simulink model "PMSM_Simulation"  (R2023a)
settings: Solver=ode23t  StartTime=0.0  StopTime=5  MaxStep=0.2  RelTol=1e-4  EnableMultiTasking=on
InitFcn:
  | p = 4;
  | Ld = 0.000425;
  | Lq = 0.00085;
  | psim = 0.119489;
  | Rs = 0.0485;
  | J = 0.00027;
  | Kpwm = 1;
  | Tsi = 0.0001;
  | h = 900;
  | 
  | L0 = (Ld+Lq)/2;
  | SMO_Kp = 100;
  | SMO_Coef =0.0001;
  | Ki_id = Ld*(h+1)/(4.5*Kpwm*(Tsi^2)*(h^2));
  | Kp_id = Ld*(h+1)/(4.5*Kpwm*Tsi*h);
  | 
  | wc =3000;
  | 
  | Ki_iq = Lq*(h+1)/(4.5*Kpwm*Tsi^2*h^2);
  | Kp_iq = Lq*(h+1)/(4.5*Kpwm*Tsi*h);
  | 
  | 
  | Kp_Spd = pi*J/(300*p*psim*Tsi)
  | Ki_Spd = pi*J/(6000*p*psim*Tsi^2)
  | 
  | DeadTime = 2e-6;
  | 
  | Udc = 650;
model workspace (MAT data in the model file):
  KfDeadCompen_CpPeriodTimesT_NULL : Simulink.Parameter (value not decoded)
  KfMDCC_InvParkCpPeriodTimesT_NULL : Simulink.Parameter (value not decoded)
values from neighbouring files (symbols this model uses):
  KfDeadCompen_SetDeltaTime_us = myPackage.Parameter    [DeadCompen.m]
  VbDeadComp_SwtUseIsttrDes_flg = myPackage.Parameter    [DeadCompen.m]
  VfDeadCompen_agIPredAdpr_C = myPackage.Parameter    [DeadCompen.m]
  VfDeadCompen_ISttrDdeThdSwt_A = myPackage.Parameter    [DeadCompen.m]
  VfDeadCompen_ISttrIgbtThdSwt_A = myPackage.Parameter    [DeadCompen.m]
  VfDeadCompen_rDdeISttrHi_R = myPackage.Parameter    [DeadCompen.m]
  VfDeadCompen_rDdeISttrLo_R = myPackage.Parameter    [DeadCompen.m]
  VfDeadCompen_rIgbtISttrHi_R = myPackage.Parameter    [DeadCompen.m]
  VfDeadCompen_rIgbtISttrLo_R = myPackage.Parameter    [DeadCompen.m]
  VfDeadCompen_uDdeISttrHi_V = myPackage.Parameter    [DeadCompen.m]
  VfDeadCompen_uDdeISttrLo_V = myPackage.Parameter    [DeadCompen.m]
  VfDeadCompen_uIgbtISttrHi_V = myPackage.Parameter    [DeadCompen.m]
  VfDeadCompen_uIgbtISttrLo_V = myPackage.Parameter    [DeadCompen.m]
symbols that are objects in the model workspace (value not decoded): KfDeadCompen_CpPeriodTimesT_NULL, KfMDCC_InvParkCpPeriodTimesT_NULL
undefined symbols (not defined in the file or in its folder): DiscIntNeverNeededParam, TableDeadTime_us, TableDeadTimeLookUpCur_A, VuDeadCompen_agIPredAdpr_C
libraries: simulink x23, mcbcontrolslib x11, mcbplantlib x1, spsCurrentMeasurementLib x1, spsDCVoltageSourceLib x1, spsMultimeterLib x1, spsPermanentMagnetSynchronousMachineLib x1, eePmsmCurrentController x1, spsThreePhaseVIMeasurementLib x1, spsUniversalBridgeLib x1, spspowerguiLib x1
(part 3 of 4)

== system PMSM_Simulation/Subsystem/Subsystem/Subsystem2/Subsystem2/Subsystem3 ==
  eMtrSpd_rads : Inport
  eMtrPos_NULL : Inport  Port=2
  VfPwmFreq_Hz : Inport  Port=3
  Isd_A : Inport  Port=4
  Isq_A : Inport  Port=5
  Add : Sum  Inputs=+++
  Constant2 : Constant  Value=2*pi  OutDataTypeStr=single
  Constant3 : Constant  Value=pi/6  OutDataTypeStr=single
  Constant4 : Constant  Value=pi/3  OutDataTypeStr=single
  Data Type Conversion : DataTypeConversion  OutDataTypeStr=uint8  SaturateOnIntegerOverflow=off  RndMeth=Floor
  Divide : Product  Inputs=*/
  Mod : Math  Operator=mod
  Subsystem1 : Subsystem
  Subsystem2 : Subsystem
  PreMtrPos : Outport
  Select_N : Outport  Port=2
  wires:
  Constant3/1 -> Add/3
  Mod/1 -> Divide/1
  Subsystem2/1(PreMtrPos) -> PreMtrPos/1, Add/1
  Constant2/1 -> Mod/2
  eMtrPos_NULL/1 -> Subsystem2/2(eMtrPos_NULL)
  Add/1 -> Mod/1
  Subsystem1/1(agIsE) -> Add/2
  Divide/1 -> Data Type Conversion/1
  Constant4/1 -> Divide/2
  Data Type Conversion/1 -> Select_N/1
  Isq_A/1 -> Subsystem1/2(Isq_A)
  Isd_A/1 -> Subsystem1/1(Isd_A)
  VfPwmFreq_Hz/1 -> Subsystem2/3(VfPwmFreq_Hz)
  eMtrSpd_rads/1 -> Subsystem2/1(eMtrSpd_rads)

== system PMSM_Simulation/Subsystem/Subsystem/Subsystem4/Subsystem1/Subsystem ==
  In1 : Inport
  Compare To Constant : simulink/Logic and Bit Operations/Compare To Constant  relop=>=  const=0  OutDataTypeStr=boolean
  Constant1 : Constant  Value=0
  Switch : Switch  Criteria=u2 > Threshold  SaturateOnIntegerOverflow=off  InputSameDT=off
  Out1 : Outport
  wires:
  In1/1 -> Switch/1, Compare To Constant/1
  Constant1/1 -> Switch/3
  Compare To Constant/1 -> Switch/2
  Switch/1 -> Out1/1

== system PMSM_Simulation/Subsystem/Subsystem/Subsystem4/Subsystem2/Subsystem ==
  In1 : Inport
  Compare To Constant : simulink/Logic and Bit Operations/Compare To Constant  relop=>=  const=0  OutDataTypeStr=boolean
  Constant1 : Constant  Value=0
  Switch : Switch  Criteria=u2 > Threshold  SaturateOnIntegerOverflow=off  InputSameDT=off
  Out1 : Outport
  wires:
  In1/1 -> Switch/1, Compare To Constant/1
  Constant1/1 -> Switch/3
  Compare To Constant/1 -> Switch/2
  Switch/1 -> Out1/1

== system PMSM_Simulation/Subsystem/Subsystem/Subsystem4/Subsystem3/Subsystem ==
  In1 : Inport
  Compare To Constant : simulink/Logic and Bit Operations/Compare To Constant  relop=>=  const=0  OutDataTypeStr=boolean
  Constant1 : Constant  Value=0
  Switch : Switch  Criteria=u2 > Threshold  SaturateOnIntegerOverflow=off  InputSameDT=off
  Out1 : Outport
  wires:
  In1/1 -> Switch/1, Compare To Constant/1
  Constant1/1 -> Switch/3
  Compare To Constant/1 -> Switch/2
  Switch/1 -> Out1/1

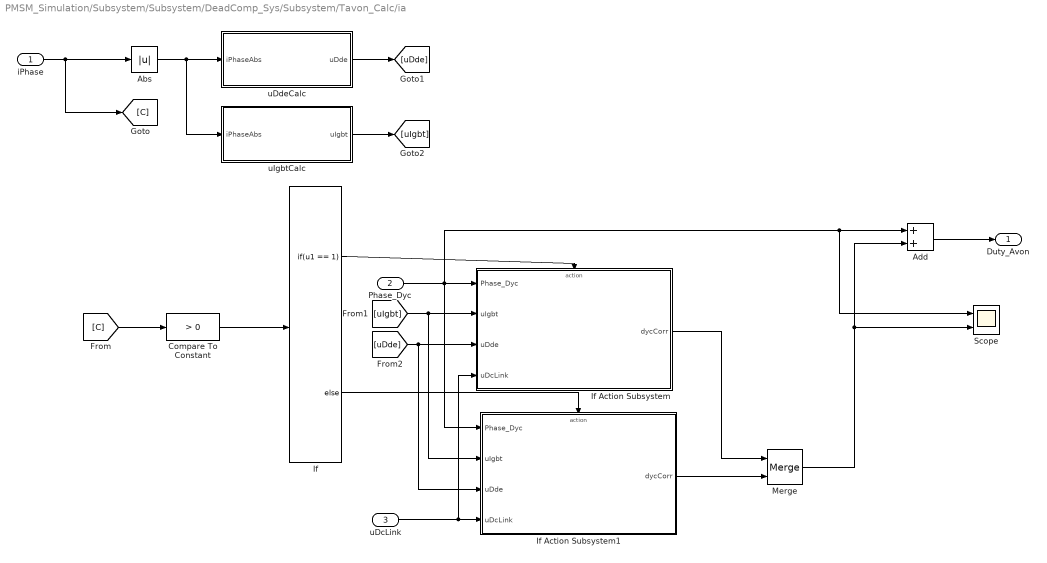
== system PMSM_Simulation/Subsystem/Subsystem/DeadComp_Sys/Subsystem/Tavon_Calc/ia ==
  iPhase : Inport
  Phase_Dyc : Inport  Port=2
  uDcLink : Inport  Port=3
  Abs : Abs  SaturateOnIntegerOverflow=off
  Add : Sum
  Compare To Constant : simulink/Logic and Bit Operations/Compare To Constant  relop=>  const=0  OutDataTypeStr=boolean
  If : If  IfExpression=u1 == 1
  If Action Subsystem : Subsystem  TreatAsAtomicUnit=on
  If Action Subsystem1 : Subsystem  TreatAsAtomicUnit=on
  Merge : Merge
  Scope : Scope  NumInputPorts=2
  uDdeCalc : Subsystem
  uIgbtCalc : Subsystem
  "Duty_Avon " : Outport
  wires:
  iPhase/1 -> [C], Abs/1
  Abs/1 -> uIgbtCalc/1(iPhaseAbs), uDdeCalc/1(iPhaseAbs)
  uDdeCalc/1(uDde) -> [uDde]
  uIgbtCalc/1(uIgbt) -> [uIgbt]
  [C] -> Compare To Constant/1
  Compare To Constant/1 -> If/1
  If/1 -> If Action Subsystem/Action
  If/2 -> If Action Subsystem1/Action
  [uIgbt] -> If Action Subsystem1/2(uIgbt), If Action Subsystem/2(uIgbt)
  [uDde] -> If Action Subsystem1/3(uDde), If Action Subsystem/3(uDde)
  Phase_Dyc/1 -> Scope/1, Add/1, If Action Subsystem1/1(Phase_Dyc), If Action Subsystem/1(Phase_Dyc)
  uDcLink/1 -> If Action Subsystem/4(uDcLink), If Action Subsystem1/4(uDcLink)
  If Action Subsystem1/1("dycCorr ") -> Merge/2
  If Action Subsystem/1("dycCorr ") -> Merge/1
  Add/1 -> "Duty_Avon "/1
  Merge/1 -> Scope/2, Add/2

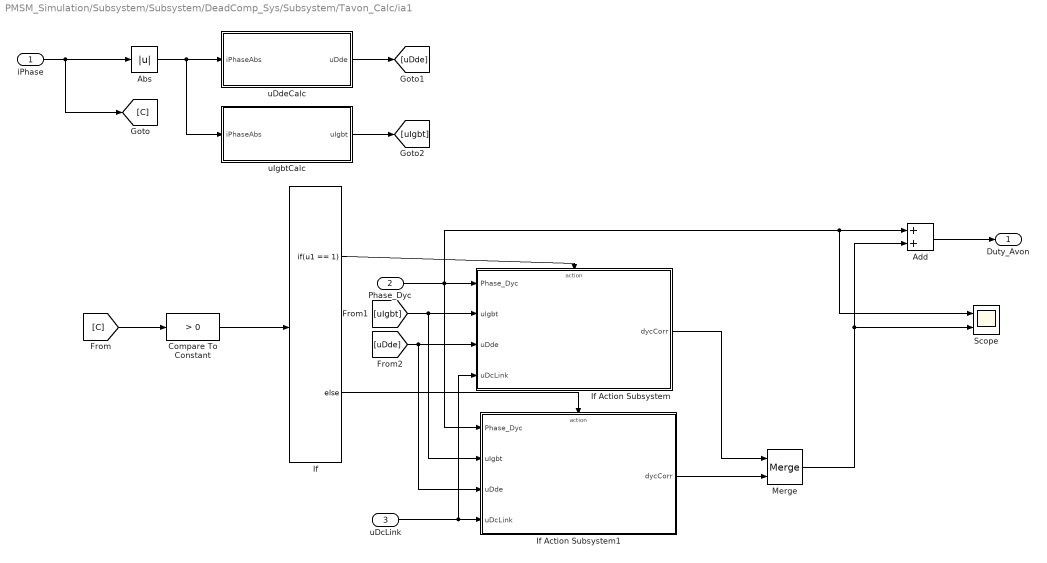
== system PMSM_Simulation/Subsystem/Subsystem/DeadComp_Sys/Subsystem/Tavon_Calc/ia1 ==
  iPhase : Inport
  Phase_Dyc : Inport  Port=2
  uDcLink : Inport  Port=3
  Abs : Abs  SaturateOnIntegerOverflow=off
  Add : Sum
  Compare To Constant : simulink/Logic and Bit Operations/Compare To Constant  relop=>  const=0  OutDataTypeStr=boolean
  If : If  IfExpression=u1 == 1
  If Action Subsystem : Subsystem  TreatAsAtomicUnit=on
  If Action Subsystem1 : Subsystem  TreatAsAtomicUnit=on
  Merge : Merge
  Scope : Scope  NumInputPorts=2
  uDdeCalc : Subsystem
  uIgbtCalc : Subsystem
  "Duty_Avon " : Outport
  wires:
  iPhase/1 -> [C], Abs/1
  Abs/1 -> uIgbtCalc/1(iPhaseAbs), uDdeCalc/1(iPhaseAbs)
  uDdeCalc/1(uDde) -> [uDde]
  uIgbtCalc/1(uIgbt) -> [uIgbt]
  [C] -> Compare To Constant/1
  Compare To Constant/1 -> If/1
  If/1 -> If Action Subsystem/Action
  If/2 -> If Action Subsystem1/Action
  [uIgbt] -> If Action Subsystem1/2(uIgbt), If Action Subsystem/2(uIgbt)
  [uDde] -> If Action Subsystem1/3(uDde), If Action Subsystem/3(uDde)
  Phase_Dyc/1 -> Scope/1, Add/1, If Action Subsystem1/1(Phase_Dyc), If Action Subsystem/1(Phase_Dyc)
  uDcLink/1 -> If Action Subsystem/4(uDcLink), If Action Subsystem1/4(uDcLink)
  If Action Subsystem1/1("dycCorr ") -> Merge/2
  If Action Subsystem/1("dycCorr ") -> Merge/1
  Add/1 -> "Duty_Avon "/1
  Merge/1 -> Scope/2, Add/2

== system PMSM_Simulation/Subsystem/Subsystem/DeadComp_Sys/Subsystem/Tavon_Calc/ia2 ==
  iPhase : Inport
  Phase_Dyc : Inport  Port=2
  uDcLink : Inport  Port=3
  Abs : Abs  SaturateOnIntegerOverflow=off
  Add : Sum
  Compare To Constant : simulink/Logic and Bit Operations/Compare To Constant  relop=>  const=0  OutDataTypeStr=boolean
  If : If  IfExpression=u1 == 1
  If Action Subsystem : Subsystem  TreatAsAtomicUnit=on
  If Action Subsystem1 : Subsystem  TreatAsAtomicUnit=on
  Merge : Merge
  Scope : Scope  NumInputPorts=2
  uDdeCalc : Subsystem
  uIgbtCalc : Subsystem
  "Duty_Avon " : Outport
  wires:
  iPhase/1 -> [C], Abs/1
  Abs/1 -> uIgbtCalc/1(iPhaseAbs), uDdeCalc/1(iPhaseAbs)
  uDdeCalc/1(uDde) -> [uDde]
  uIgbtCalc/1(uIgbt) -> [uIgbt]
  [C] -> Compare To Constant/1
  Compare To Constant/1 -> If/1
  If/1 -> If Action Subsystem/Action
  If/2 -> If Action Subsystem1/Action
  [uIgbt] -> If Action Subsystem1/2(uIgbt), If Action Subsystem/2(uIgbt)
  [uDde] -> If Action Subsystem1/3(uDde), If Action Subsystem/3(uDde)
  Phase_Dyc/1 -> Scope/1, Add/1, If Action Subsystem1/1(Phase_Dyc), If Action Subsystem/1(Phase_Dyc)
  uDcLink/1 -> If Action Subsystem/4(uDcLink), If Action Subsystem1/4(uDcLink)
  If Action Subsystem1/1("dycCorr ") -> Merge/2
  If Action Subsystem/1("dycCorr ") -> Merge/1
  Add/1 -> "Duty_Avon "/1
  Merge/1 -> Scope/2, Add/2

== system PMSM_Simulation/Subsystem/Subsystem/DeadComp_Sys/Subsystem2/Subsystem3/Subsystem1 ==
  Isd_A : Inport
  Isq_A : Inport  Port=2
  Add : Sum
  Atan2 : Trigonometry  Operator=atan2
  Constant : Constant  Value=2*pi  OutDataTypeStr=single
  Switch : Switch  Criteria=u2 > Threshold  SaturateOnIntegerOverflow=off  InputSameDT=off
  agIsE : Outport
  wires:
  Isd_A/1 -> Atan2/2
  Isq_A/1 -> Atan2/1
  Atan2/1 -> Add/1, Switch/1, Switch/2
  Switch/1 -> agIsE/1
  Add/1 -> Switch/3
  Constant/1 -> Add/2

== system PMSM_Simulation/Subsystem/Subsystem/DeadComp_Sys/Subsystem2/Subsystem3/Subsystem2 ==
  eMtrSpd_rads : Inport
  eMtrPos_NULL : Inport  Port=2
  VfPwmFreq_Hz : Inport  Port=3
  Add : Sum  Inputs=+++
  Constant : Constant  Value=VuDeadCompen_agIPredAdpr_C
  Gain : Gain  Gain=2*pi/4095
  Gain1 : Gain  Gain=-1
  Gain2 : Gain  Gain=2*pi/4095
  Product : Product
  Subsystem : Subsystem
  Switch : Switch  Criteria=u2 > Threshold  SaturateOnIntegerOverflow=off  InputSameDT=off
  PreMtrPos : Outport
  wires:
  VfPwmFreq_Hz/1 -> Subsystem/1(VfPwmFreq_Hz)
  Subsystem/1(TimeComp) -> Product/2
  eMtrPos_NULL/1 -> Gain/1
  Product/1 -> Add/2
  Gain/1 -> Add/3
  Add/1 -> PreMtrPos/1
  eMtrSpd_rads/1 -> Product/1, Switch/2
  Constant/1 -> Gain2/1
  Gain1/1 -> Switch/3
  Gain2/1 -> Gain1/1, Switch/1
  Switch/1 -> Add/1

== system PMSM_Simulation/Subsystem/Subsystem/SVM_PU/T1_T2_Calc/Subsystem1/Enabled Subsystem ==
  Z : Inport
  Y : Inport  Port=2
  Action Port : ActionPort  ActionPortLabel=case [ 1 ]:
  T4 : Outport
  T6 : Outport  Port=2
  wires:
  Z/1 -> T4/1
  Y/1 -> T6/1

== system PMSM_Simulation/Subsystem/Subsystem/SVM_PU/T1_T2_Calc/Subsystem1/Enabled Subsystem1 ==
  Y : Inport
  X : Inport  Port=2
  Action Port : ActionPort  ActionPortLabel=case [ 2 ]:
  Gain : Gain  Gain=-1
  T4 : Outport
  T6 : Outport  Port=2
  wires:
  Y/1 -> T4/1
  Gain/1 -> T6/1
  X/1 -> Gain/1

== system PMSM_Simulation/Subsystem/Subsystem/SVM_PU/T1_T2_Calc/Subsystem1/Enabled Subsystem2 ==
  Z : Inport
  X : Inport  Port=2
  Action Port : ActionPort  ActionPortLabel=case [ 3 ]:
  Gain : Gain  Gain=-1
  T4 : Outport
  T6 : Outport  Port=2
  wires:
  Z/1 -> Gain/1
  X/1 -> T6/1
  Gain/1 -> T4/1

== system PMSM_Simulation/Subsystem/Subsystem/SVM_PU/T1_T2_Calc/Subsystem1/Enabled Subsystem3 ==
  X : Inport
  Z : Inport  Port=2
  Action Port : ActionPort  ActionPortLabel=case [ 4 ]:
  Gain : Gain  Gain=-1
  T4 : Outport
  T6 : Outport  Port=2
  wires:
  X/1 -> Gain/1
  Z/1 -> T6/1
  Gain/1 -> T4/1

== system PMSM_Simulation/Subsystem/Subsystem/SVM_PU/T1_T2_Calc/Subsystem1/Enabled Subsystem4 ==
  X : Inport
  Y : Inport  Port=2
  Action Port : ActionPort  ActionPortLabel=case [ 5 ]:
  Gain : Gain  Gain=-1
  T4 : Outport
  T6 : Outport  Port=2
  wires:
  Y/1 -> Gain/1
  X/1 -> T4/1
  Gain/1 -> T6/1

== system PMSM_Simulation/Subsystem/Subsystem/SVM_PU/T1_T2_Calc/Subsystem1/Enabled Subsystem5 ==
  Y : Inport
  Z : Inport  Port=2
  Action Port : ActionPort  ActionPortLabel=case [ 6 ]:
  Gain : Gain  Gain=-1
  Gain1 : Gain  Gain=-1
  T4 : Outport
  T6 : Outport  Port=2
  wires:
  Y/1 -> Gain/1
  Z/1 -> Gain1/1
  Gain/1 -> T4/1
  Gain1/1 -> T6/1

== system PMSM_Simulation/Subsystem/Subsystem/SVM_PU/T1_T2_Calc/Subsystem1/Enabled Subsystem6 ==
  Y : Inport
  Z : Inport  Port=2
  Action Port : ActionPort  ActionPortLabel=default:
  Gain : Gain  Gain=-1
  Gain1 : Gain  Gain=-1
  T4 : Outport
  T6 : Outport  Port=2
  wires:
  Y/1 -> Gain/1
  Z/1 -> Gain1/1
  Gain/1 -> T4/1
  Gain1/1 -> T6/1

== system PMSM_Simulation/Subsystem/Subsystem/SVM_PU/T1_T2_Calc/Subsystem2/If Action Subsystem ==
  Bus_T4T6 : Inport
  Action Port : ActionPort  ActionPortLabel=else
  Bus Selector : BusSelector  OutputSignals=T4,T6
  Signal Copy1 : SignalConversion  OverrideOpt=off
  Signal Copy2 : SignalConversion  OverrideOpt=off
  T1 : Outport
  T2 : Outport  Port=2
  wires:
  Bus_T4T6/1 -> Bus Selector/1
  Bus Selector/1 -> Signal Copy1/1  "<T4>"
  Bus Selector/2 -> Signal Copy2/1  "<T6>"
  Signal Copy1/1 -> T1/1
  Signal Copy2/1 -> T2/1

== system PMSM_Simulation/Subsystem/Subsystem/SVM_PU/T1_T2_Calc/Subsystem2/If Action Subsystem1 ==
  Bus_T4T6 : Inport
  Action Port : ActionPort  ActionPortLabel=elseif(u1 > 1)
  Add : Sum
  Bus Selector : BusSelector  OutputSignals=T4,T6
  Divide : Product  Inputs=*/
  Divide1 : Product  Inputs=/*
  T1 : Outport
  T2 : Outport  Port=2
  wires:
  Bus_T4T6/1 -> Bus Selector/1
  Bus Selector/1 -> Divide/1, Add/1  "<T4>"
  Bus Selector/2 -> Divide1/2, Add/2  "<T6>"
  Add/1 -> Divide1/1, Divide/2
  Divide/1 -> T1/1  "T1"
  Divide1/1 -> T2/1  "T2"

== system PMSM_Simulation/Subsystem/Subsystem/SVM_PU/T1_T2_Calc/Subsystem2/If Action Subsystem2 ==
  Bus_T4T6 : Inport
  Action Port : ActionPort  ActionPortLabel=if(u1 > 1.154 )
  Add1 : Sum
  Add2 : Sum  Inputs=++-
  Bus Selector1 : BusSelector  OutputSignals=T4,T6
  Constant : Constant  Value=1.154  OutDataTypeStr=single
  Divide : Product  Inputs=*/
  Divide1 : Product  Inputs=/*
  If Action Subsystem2 : Subsystem  TreatAsAtomicUnit=on
  If Action Subsystem3 : Subsystem  TreatAsAtomicUnit=on
  If1 : If  IfExpression=u1 ~= 0
  Merge2 : Merge
  Merge3 : Merge
  Relational Operator1 : RelationalOperator  OutDataTypeStr=boolean  RndMeth=Simplest  InputSameDT=off
  T1 : Outport
  T2 : Outport  Port=2
  wires:
  Bus_T4T6/1 -> Bus Selector1/1
  Bus Selector1/2 -> Divide1/2, Add2/2, Add1/2  "<T6>"
  Divide/1 -> [T4_m], Relational Operator1/1  "T4_m"
  Bus Selector1/1 -> Divide/1, Add2/1, Add1/1  "<T4>"
  Divide1/1 -> [T6_m], Relational Operator1/2  "T6_m"
  Add1/1 -> Divide1/1, Divide/2
  Relational Operator1/1 -> If1/1
  Constant/1 -> Add2/3
  Add2/1 -> If Action Subsystem2/3(delta), If Action Subsystem3/3(delta)  "delta"
  If1/1 -> If Action Subsystem2/Action
  If1/2 -> If Action Subsystem3/Action
  If Action Subsystem2/1(T1) -> Merge2/1
  If Action Subsystem3/1(T1) -> Merge2/2
  If Action Subsystem3/2(T2) -> Merge3/2
  If Action Subsystem2/2(T2) -> Merge3/1
  Merge2/1 -> T1/1  "T1"
  Merge3/1 -> T2/1  "T2"
  [T4_m] -> If Action Subsystem3/1(T4_m), If Action Subsystem2/1(T4_m)
  [T6_m] -> If Action Subsystem3/2(T6_m), If Action Subsystem2/2(T6_m)

== system PMSM_Simulation/Subsystem/Subsystem/Subsystem2/Subsystem/DutyErr_Calc/PhaseU ==
  Bus_DutyAvon : Inport
  Bus_DeltaTimeOnOffDuty : Inport  Port=2
  DeadTimeDuty : Inport  Port=3
  Add : Sum  Inputs=+-+
  Bus Selector : BusSelector  OutputSignals=DutyAvon_U
  Bus Selector1 : BusSelector  OutputSignals=DeltaTimeOnOffU_NULL
  DutyCompensate_U : Outport
  wires:
  Bus_DutyAvon/1 -> Bus Selector/1
  Bus_DeltaTimeOnOffDuty/1 -> Bus Selector1/1
  Bus Selector1/1 -> Add/2  "<DeltaTimeOnOffU_NULL>"
  Bus Selector/1 -> Add/1  "<DutyAvon_U>"
  DeadTimeDuty/1 -> Add/3
  Add/1 -> DutyCompensate_U/1

== system PMSM_Simulation/Subsystem/Subsystem/Subsystem2/Subsystem/DutyErr_Calc/PhaseV ==
  Bus_DutyAvon : Inport
  Bus_DeltaTimeOnOffDuty : Inport  Port=2
  DeadTimeDuty : Inport  Port=3
  Add : Sum  Inputs=+++
  Bus Selector : BusSelector  OutputSignals=DutyAvon_V
  Bus Selector1 : BusSelector  OutputSignals=DeltaTimeOnOffV_NULL
  DutyCompensate_V : Outport
  wires:
  Bus_DutyAvon/1 -> Bus Selector/1
  Bus_DeltaTimeOnOffDuty/1 -> Bus Selector1/1
  Bus Selector1/1 -> Add/2  "<DeltaTimeOnOffV_NULL>"
  Bus Selector/1 -> Add/1  "<DutyAvon_V>"
  DeadTimeDuty/1 -> Add/3
  Add/1 -> DutyCompensate_V/1

== system PMSM_Simulation/Subsystem/Subsystem/Subsystem2/Subsystem/DutyErr_Calc/PhaseW ==
  Bus_DutyAvon : Inport
  Bus_DeltaTimeOnOffDuty : Inport  Port=2
  DeadTimeDuty : Inport  Port=3
  Add : Sum  Inputs=+++
  Bus Selector : BusSelector  OutputSignals=DutyAvon_W
  Bus Selector1 : BusSelector  OutputSignals=DeltaTimeOnOffW_NULL
  DutyCompensate_W : Outport
  wires:
  Bus_DutyAvon/1 -> Bus Selector/1
  Bus_DeltaTimeOnOffDuty/1 -> Bus Selector1/1
  Bus Selector1/1 -> Add/2  "<DeltaTimeOnOffW_NULL>"
  Bus Selector/1 -> Add/1  "<DutyAvon_W>"
  DeadTimeDuty/1 -> Add/3
  Add/1 -> DutyCompensate_W/1

== system PMSM_Simulation/Subsystem/Subsystem/Subsystem2/Subsystem/Tavon_Calc/ia ==
  iPhase : Inport
  Phase_Dyc : Inport  Port=2
  uDcLink : Inport  Port=3
  Abs : Abs  SaturateOnIntegerOverflow=off
  Add : Sum
  Compare To Constant : simulink/Logic and Bit Operations/Compare To Constant  relop=>  const=0  OutDataTypeStr=boolean
  If : If  IfExpression=u1 == 1
  If Action Subsystem : Subsystem  TreatAsAtomicUnit=on
  If Action Subsystem1 : Subsystem  TreatAsAtomicUnit=on
  Merge : Merge
  Scope : Scope  NumInputPorts=2
  uDdeCalc : Subsystem
  uIgbtCalc : Subsystem
  "Duty_Avon " : Outport
  wires:
  iPhase/1 -> [C], Abs/1
  Abs/1 -> uIgbtCalc/1(iPhaseAbs), uDdeCalc/1(iPhaseAbs)
  uDdeCalc/1(uDde) -> [uDde]
  uIgbtCalc/1(uIgbt) -> [uIgbt]
  [C] -> Compare To Constant/1
  Compare To Constant/1 -> If/1
  If/1 -> If Action Subsystem/Action
  If/2 -> If Action Subsystem1/Action
  [uIgbt] -> If Action Subsystem1/2(uIgbt), If Action Subsystem/2(uIgbt)
  [uDde] -> If Action Subsystem1/3(uDde), If Action Subsystem/3(uDde)
  Phase_Dyc/1 -> Scope/1, Add/1, If Action Subsystem1/1(Phase_Dyc), If Action Subsystem/1(Phase_Dyc)
  uDcLink/1 -> If Action Subsystem/4(uDcLink), If Action Subsystem1/4(uDcLink)
  If Action Subsystem1/1("dycCorr ") -> Merge/2
  If Action Subsystem/1("dycCorr ") -> Merge/1
  Add/1 -> "Duty_Avon "/1
  Merge/1 -> Scope/2, Add/2

== system PMSM_Simulation/Subsystem/Subsystem/Subsystem2/Subsystem/Tavon_Calc/ia1 ==
  iPhase : Inport
  Phase_Dyc : Inport  Port=2
  uDcLink : Inport  Port=3
  Abs : Abs  SaturateOnIntegerOverflow=off
  Add : Sum
  Compare To Constant : simulink/Logic and Bit Operations/Compare To Constant  relop=>  const=0  OutDataTypeStr=boolean
  If : If  IfExpression=u1 == 1
  If Action Subsystem : Subsystem  TreatAsAtomicUnit=on
  If Action Subsystem1 : Subsystem  TreatAsAtomicUnit=on
  Merge : Merge
  Scope : Scope  NumInputPorts=2
  uDdeCalc : Subsystem
  uIgbtCalc : Subsystem
  "Duty_Avon " : Outport
  wires:
  iPhase/1 -> [C], Abs/1
  Abs/1 -> uIgbtCalc/1(iPhaseAbs), uDdeCalc/1(iPhaseAbs)
  uDdeCalc/1(uDde) -> [uDde]
  uIgbtCalc/1(uIgbt) -> [uIgbt]
  [C] -> Compare To Constant/1
  Compare To Constant/1 -> If/1
  If/1 -> If Action Subsystem/Action
  If/2 -> If Action Subsystem1/Action
  [uIgbt] -> If Action Subsystem1/2(uIgbt), If Action Subsystem/2(uIgbt)
  [uDde] -> If Action Subsystem1/3(uDde), If Action Subsystem/3(uDde)
  Phase_Dyc/1 -> Scope/1, Add/1, If Action Subsystem1/1(Phase_Dyc), If Action Subsystem/1(Phase_Dyc)
  uDcLink/1 -> If Action Subsystem/4(uDcLink), If Action Subsystem1/4(uDcLink)
  If Action Subsystem1/1("dycCorr ") -> Merge/2
  If Action Subsystem/1("dycCorr ") -> Merge/1
  Add/1 -> "Duty_Avon "/1
  Merge/1 -> Scope/2, Add/2

== system PMSM_Simulation/Subsystem/Subsystem/Subsystem2/Subsystem/Tavon_Calc/ia2 ==
  iPhase : Inport
  Phase_Dyc : Inport  Port=2
  uDcLink : Inport  Port=3
  Abs : Abs  SaturateOnIntegerOverflow=off
  Add : Sum
  Compare To Constant : simulink/Logic and Bit Operations/Compare To Constant  relop=>  const=0  OutDataTypeStr=boolean
  If : If  IfExpression=u1 == 1
  If Action Subsystem : Subsystem  TreatAsAtomicUnit=on
  If Action Subsystem1 : Subsystem  TreatAsAtomicUnit=on
  Merge : Merge
  Scope : Scope  NumInputPorts=2
  uDdeCalc : Subsystem
  uIgbtCalc : Subsystem
  "Duty_Avon " : Outport
  wires:
  iPhase/1 -> [C], Abs/1
  Abs/1 -> uIgbtCalc/1(iPhaseAbs), uDdeCalc/1(iPhaseAbs)
  uDdeCalc/1(uDde) -> [uDde]
  uIgbtCalc/1(uIgbt) -> [uIgbt]
  [C] -> Compare To Constant/1
  Compare To Constant/1 -> If/1
  If/1 -> If Action Subsystem/Action
  If/2 -> If Action Subsystem1/Action
  [uIgbt] -> If Action Subsystem1/2(uIgbt), If Action Subsystem/2(uIgbt)
  [uDde] -> If Action Subsystem1/3(uDde), If Action Subsystem/3(uDde)
  Phase_Dyc/1 -> Scope/1, Add/1, If Action Subsystem1/1(Phase_Dyc), If Action Subsystem/1(Phase_Dyc)
  uDcLink/1 -> If Action Subsystem/4(uDcLink), If Action Subsystem1/4(uDcLink)
  If Action Subsystem1/1("dycCorr ") -> Merge/2
  If Action Subsystem/1("dycCorr ") -> Merge/1
  Add/1 -> "Duty_Avon "/1
  Merge/1 -> Scope/2, Add/2

== system PMSM_Simulation/Subsystem/Subsystem/Subsystem2/Subsystem2/Subsystem3/Subsystem1 ==
  Isd_A : Inport
  Isq_A : Inport  Port=2
  Add : Sum
  Atan2 : Trigonometry  Operator=atan2
  Constant : Constant  Value=2*pi  OutDataTypeStr=single
  Switch : Switch  Criteria=u2 > Threshold  SaturateOnIntegerOverflow=off  InputSameDT=off
  agIsE : Outport
  wires:
  Isd_A/1 -> Atan2/2
  Isq_A/1 -> Atan2/1
  Atan2/1 -> Add/1, Switch/1, Switch/2
  Switch/1 -> agIsE/1
  Add/1 -> Switch/3
  Constant/1 -> Add/2

== system PMSM_Simulation/Subsystem/Subsystem/Subsystem2/Subsystem2/Subsystem3/Subsystem2 ==
  eMtrSpd_rads : Inport
  eMtrPos_NULL : Inport  Port=2
  VfPwmFreq_Hz : Inport  Port=3
  Add : Sum  Inputs=+++
  Constant : Constant  Value=VfDeadCompen_agIPredAdpr_C
  Gain : Gain  Gain=2*pi/4095
  Gain1 : Gain  Gain=-1
  Gain2 : Gain  Gain=2*pi/4095
  Product : Product
  Subsystem : Subsystem
  Switch : Switch  Criteria=u2 > Threshold  SaturateOnIntegerOverflow=off  InputSameDT=off
  PreMtrPos : Outport
  wires:
  VfPwmFreq_Hz/1 -> Subsystem/1(VfPwmFreq_Hz)
  Subsystem/1(TimeComp) -> Product/2
  eMtrPos_NULL/1 -> Gain/1
  Product/1 -> Add/2
  Gain/1 -> Add/3
  Add/1 -> PreMtrPos/1
  eMtrSpd_rads/1 -> Product/1, Switch/2
  Constant/1 -> Gain2/1
  Gain1/1 -> Switch/3
  Gain2/1 -> Gain1/1, Switch/1
  Switch/1 -> Add/1

== system PMSM_Simulation/Subsystem/Subsystem/DeadComp_Sys/Subsystem/Tavon_Calc/ia/If Action Subsystem ==
  Phase_Dyc : Inport
  uIgbt : Inport  Port=2
  uDde : Inport  Port=3
  uDcLink : Inport  Port=4
  Action Port : ActionPort
  Add : Sum  Inputs=-+
  Add1 : Sum  Inputs=+-
  Add2 : Sum  Inputs=--+
  Constant : Constant  OutDataTypeStr=single
  Divide : Product  Inputs=*/
  Product : Product
  Product1 : Product
  "dycCorr " : Outport
  wires:
  Phase_Dyc/1 -> Product/1, Add/1
  uIgbt/1 -> Product/2, Add2/1
  uDde/1 -> Add2/2, Product1/2
  Add/1 -> Product1/1
  Constant/1 -> Add/2
  Product/1 -> Add1/1
  Product1/1 -> Add1/2
  uDcLink/1 -> Add2/3
  Add1/1 -> Divide/1
  Add2/1 -> Divide/2
  Divide/1 -> "dycCorr "/1

== system PMSM_Simulation/Subsystem/Subsystem/DeadComp_Sys/Subsystem/Tavon_Calc/ia/If Action Subsystem1 ==
  Phase_Dyc : Inport
  uIgbt : Inport  Port=2
  uDde : Inport  Port=3
  uDcLink : Inport  Port=4
  Action Port : ActionPort
  Add : Sum  Inputs=-+
  Add1 : Sum  Inputs=+-
  Add2 : Sum  Inputs=--+
  Constant : Constant  OutDataTypeStr=single
  Divide : Product  Inputs=*/
  Product : Product
  Product1 : Product
  "dycCorr " : Outport
  wires:
  Phase_Dyc/1 -> Product/1, Add/1
  uDde/1 -> Add2/1, Product/2
  uIgbt/1 -> Add2/2, Product1/2
  Add/1 -> Product1/1
  Constant/1 -> Add/2
  Product/1 -> Add1/1
  Product1/1 -> Add1/2
  uDcLink/1 -> Add2/3
  Add1/1 -> Divide/1
  Add2/1 -> Divide/2
  Divide/1 -> "dycCorr "/1

== system PMSM_Simulation/Subsystem/Subsystem/DeadComp_Sys/Subsystem/Tavon_Calc/ia/uDdeCalc ==
  iPhaseAbs : Inport
  Compare To Constant : simulink/Logic and Bit Operations/Compare To Constant  relop=<  const=VfDeadCompen_ISttrDdeThdSwt_A  OutDataTypeStr=boolean
  From : From
  From1 : From
  Goto : Goto
  If : If  IfExpression=u1 == 1
  If Action Subsystem : Subsystem  TreatAsAtomicUnit=on
  If Action Subsystem1 : Subsystem  TreatAsAtomicUnit=on
  Merge : Merge
  uDde : Outport
  wires:
  iPhaseAbs/1 -> Goto/1, Compare To Constant/1
  If/2 -> If Action Subsystem1/Action
  Merge/1 -> uDde/1
  If/1 -> If Action Subsystem/Action
  If Action Subsystem/1(UDde) -> Merge/1
  Compare To Constant/1 -> If/1
  If Action Subsystem1/1(UDde) -> Merge/2
  From1/1 -> If Action Subsystem/1(iPhaseAbs)
  From/1 -> If Action Subsystem1/1(iPhaseAbs)

== system PMSM_Simulation/Subsystem/Subsystem/DeadComp_Sys/Subsystem/Tavon_Calc/ia/uIgbtCalc ==
  iPhaseAbs : Inport
  Compare To Constant : simulink/Logic and Bit Operations/Compare To Constant  relop=<  const=VfDeadCompen_ISttrIgbtThdSwt_A  OutDataTypeStr=boolean
  If : If  IfExpression=u1 == 0
  If Action Subsystem : Subsystem  TreatAsAtomicUnit=on
  If Action Subsystem1 : Subsystem  TreatAsAtomicUnit=on
  Merge : Merge
  uIgbt : Outport
  wires:
  iPhaseAbs/1 -> Compare To Constant/1, [B]
  If/2 -> If Action Subsystem1/Action
  Merge/1 -> uIgbt/1
  If/1 -> If Action Subsystem/Action
  If Action Subsystem/1(uIgbt) -> Merge/1
  Compare To Constant/1 -> If/1
  If Action Subsystem1/1(uIgbt) -> Merge/2
  [B] -> If Action Subsystem/1(iPhaseAbs)
  [B] -> If Action Subsystem1/1(iPhaseAbs)

== system PMSM_Simulation/Subsystem/Subsystem/DeadComp_Sys/Subsystem/Tavon_Calc/ia1/If Action Subsystem ==
  Phase_Dyc : Inport
  uIgbt : Inport  Port=2
  uDde : Inport  Port=3
  uDcLink : Inport  Port=4
  Action Port : ActionPort
  Add : Sum  Inputs=-+
  Add1 : Sum  Inputs=+-
  Add2 : Sum  Inputs=--+
  Constant : Constant  OutDataTypeStr=single
  Divide : Product  Inputs=*/
  Product : Product
  Product1 : Product
  "dycCorr " : Outport
  wires:
  Phase_Dyc/1 -> Product/1, Add/1
  uIgbt/1 -> Product/2, Add2/1
  uDde/1 -> Add2/2, Product1/2
  Add/1 -> Product1/1
  Constant/1 -> Add/2
  Product/1 -> Add1/1
  Product1/1 -> Add1/2
  uDcLink/1 -> Add2/3
  Add1/1 -> Divide/1
  Add2/1 -> Divide/2
  Divide/1 -> "dycCorr "/1

== system PMSM_Simulation/Subsystem/Subsystem/DeadComp_Sys/Subsystem/Tavon_Calc/ia1/If Action Subsystem1 ==
  Phase_Dyc : Inport
  uIgbt : Inport  Port=2
  uDde : Inport  Port=3
  uDcLink : Inport  Port=4
  Action Port : ActionPort
  Add : Sum  Inputs=-+
  Add1 : Sum  Inputs=+-
  Add2 : Sum  Inputs=--+
  Constant : Constant  OutDataTypeStr=single
  Divide : Product  Inputs=*/
  Product : Product
  Product1 : Product
  "dycCorr " : Outport
  wires:
  Phase_Dyc/1 -> Product/1, Add/1
  uDde/1 -> Add2/1, Product/2
  uIgbt/1 -> Add2/2, Product1/2
  Add/1 -> Product1/1
  Constant/1 -> Add/2
  Product/1 -> Add1/1
  Product1/1 -> Add1/2
  uDcLink/1 -> Add2/3
  Add1/1 -> Divide/1
  Add2/1 -> Divide/2
  Divide/1 -> "dycCorr "/1

== system PMSM_Simulation/Subsystem/Subsystem/DeadComp_Sys/Subsystem/Tavon_Calc/ia1/uDdeCalc ==
  iPhaseAbs : Inport
  Compare To Constant : simulink/Logic and Bit Operations/Compare To Constant  relop=<  const=VfDeadCompen_ISttrDdeThdSwt_A  OutDataTypeStr=boolean
  From : From
  From1 : From
  Goto : Goto
  If : If  IfExpression=u1 == 1
  If Action Subsystem : Subsystem  TreatAsAtomicUnit=on
  If Action Subsystem1 : Subsystem  TreatAsAtomicUnit=on
  Merge : Merge
  uDde : Outport
  wires:
  iPhaseAbs/1 -> Goto/1, Compare To Constant/1
  If/2 -> If Action Subsystem1/Action
  Merge/1 -> uDde/1
  If/1 -> If Action Subsystem/Action
  If Action Subsystem/1(UDde) -> Merge/1
  Compare To Constant/1 -> If/1
  If Action Subsystem1/1(UDde) -> Merge/2
  From1/1 -> If Action Subsystem/1(iPhaseAbs)
  From/1 -> If Action Subsystem1/1(iPhaseAbs)

== system PMSM_Simulation/Subsystem/Subsystem/DeadComp_Sys/Subsystem/Tavon_Calc/ia1/uIgbtCalc ==
  iPhaseAbs : Inport
  Compare To Constant : simulink/Logic and Bit Operations/Compare To Constant  relop=<  const=VfDeadCompen_ISttrIgbtThdSwt_A  OutDataTypeStr=boolean
  If : If  IfExpression=u1 == 0
  If Action Subsystem : Subsystem  TreatAsAtomicUnit=on
  If Action Subsystem1 : Subsystem  TreatAsAtomicUnit=on
  Merge : Merge
  uIgbt : Outport
  wires:
  iPhaseAbs/1 -> Compare To Constant/1, [B]
  If/2 -> If Action Subsystem1/Action
  Merge/1 -> uIgbt/1
  If/1 -> If Action Subsystem/Action
  If Action Subsystem/1(uIgbt) -> Merge/1
  Compare To Constant/1 -> If/1
  If Action Subsystem1/1(uIgbt) -> Merge/2
  [B] -> If Action Subsystem/1(iPhaseAbs)
  [B] -> If Action Subsystem1/1(iPhaseAbs)

== system PMSM_Simulation/Subsystem/Subsystem/DeadComp_Sys/Subsystem/Tavon_Calc/ia2/If Action Subsystem ==
  Phase_Dyc : Inport
  uIgbt : Inport  Port=2
  uDde : Inport  Port=3
  uDcLink : Inport  Port=4
  Action Port : ActionPort
  Add : Sum  Inputs=-+
  Add1 : Sum  Inputs=+-
  Add2 : Sum  Inputs=--+
  Constant : Constant  OutDataTypeStr=single
  Divide : Product  Inputs=*/
  Product : Product
  Product1 : Product
  "dycCorr " : Outport
  wires:
  Phase_Dyc/1 -> Product/1, Add/1
  uIgbt/1 -> Product/2, Add2/1
  uDde/1 -> Add2/2, Product1/2
  Add/1 -> Product1/1
  Constant/1 -> Add/2
  Product/1 -> Add1/1
  Product1/1 -> Add1/2
  uDcLink/1 -> Add2/3
  Add1/1 -> Divide/1
  Add2/1 -> Divide/2
  Divide/1 -> "dycCorr "/1

== system PMSM_Simulation/Subsystem/Subsystem/DeadComp_Sys/Subsystem/Tavon_Calc/ia2/If Action Subsystem1 ==
  Phase_Dyc : Inport
  uIgbt : Inport  Port=2
  uDde : Inport  Port=3
  uDcLink : Inport  Port=4
  Action Port : ActionPort
  Add : Sum  Inputs=-+
  Add1 : Sum  Inputs=+-
  Add2 : Sum  Inputs=--+
  Constant : Constant  OutDataTypeStr=single
  Divide : Product  Inputs=*/
  Product : Product
  Product1 : Product
  "dycCorr " : Outport
  wires:
  Phase_Dyc/1 -> Product/1, Add/1
  uDde/1 -> Add2/1, Product/2
  uIgbt/1 -> Add2/2, Product1/2
  Add/1 -> Product1/1
  Constant/1 -> Add/2
  Product/1 -> Add1/1
  Product1/1 -> Add1/2
  uDcLink/1 -> Add2/3
  Add1/1 -> Divide/1
  Add2/1 -> Divide/2
  Divide/1 -> "dycCorr "/1

== system PMSM_Simulation/Subsystem/Subsystem/DeadComp_Sys/Subsystem/Tavon_Calc/ia2/uDdeCalc ==
  iPhaseAbs : Inport
  Compare To Constant : simulink/Logic and Bit Operations/Compare To Constant  relop=<  const=VfDeadCompen_ISttrDdeThdSwt_A  OutDataTypeStr=boolean
  From : From
  From1 : From
  Goto : Goto
  If : If  IfExpression=u1 == 1
  If Action Subsystem : Subsystem  TreatAsAtomicUnit=on
  If Action Subsystem1 : Subsystem  TreatAsAtomicUnit=on
  Merge : Merge
  uDde : Outport
  wires:
  iPhaseAbs/1 -> Goto/1, Compare To Constant/1
  If/2 -> If Action Subsystem1/Action
  Merge/1 -> uDde/1
  If/1 -> If Action Subsystem/Action
  If Action Subsystem/1(UDde) -> Merge/1
  Compare To Constant/1 -> If/1
  If Action Subsystem1/1(UDde) -> Merge/2
  From1/1 -> If Action Subsystem/1(iPhaseAbs)
  From/1 -> If Action Subsystem1/1(iPhaseAbs)

== system PMSM_Simulation/Subsystem/Subsystem/DeadComp_Sys/Subsystem/Tavon_Calc/ia2/uIgbtCalc ==
  iPhaseAbs : Inport
  Compare To Constant : simulink/Logic and Bit Operations/Compare To Constant  relop=<  const=VfDeadCompen_ISttrIgbtThdSwt_A  OutDataTypeStr=boolean
  If : If  IfExpression=u1 == 0
  If Action Subsystem : Subsystem  TreatAsAtomicUnit=on
  If Action Subsystem1 : Subsystem  TreatAsAtomicUnit=on
  Merge : Merge
  uIgbt : Outport
  wires:
  iPhaseAbs/1 -> Compare To Constant/1, [B]
  If/2 -> If Action Subsystem1/Action
  Merge/1 -> uIgbt/1
  If/1 -> If Action Subsystem/Action
  If Action Subsystem/1(uIgbt) -> Merge/1
  Compare To Constant/1 -> If/1
  If Action Subsystem1/1(uIgbt) -> Merge/2
  [B] -> If Action Subsystem/1(iPhaseAbs)
  [B] -> If Action Subsystem1/1(iPhaseAbs)

== system PMSM_Simulation/Subsystem/Subsystem/DeadComp_Sys/Subsystem2/Subsystem3/Subsystem2/Subsystem ==
  VfPwmFreq_Hz : Inport
  Add5 : Sum
  KfDeadCompen_CpPeriodTimesT_NULL : Constant  Value=KfDeadCompen_CpPeriodTimesT_NULL  OutDataTypeStr=single
  KfMDCC_InvParkCpPeriodTimesT_NULL : Constant  Value=KfMDCC_InvParkCpPeriodTimesT_NULL
  Product1 : Product
  TimeComp : Outport
  wires:
  KfMDCC_InvParkCpPeriodTimesT_NULL/1 -> Add5/2
  KfDeadCompen_CpPeriodTimesT_NULL/1 -> Add5/1
  VfPwmFreq_Hz/1 -> Product1/2
  Product1/1 -> TimeComp/1
  Add5/1 -> Product1/1

== system PMSM_Simulation/Subsystem/Subsystem/SVM_PU/T1_T2_Calc/Subsystem2/If Action Subsystem2/If Action Subsystem2 ==
  T4_m : Inport
  T6_m : Inport  Port=2
  delta : Inport  Port=3
  Action Port : ActionPort  ActionPortLabel=if(u1 ~= 0)
  Add : Sum
  Add1 : Sum  Inputs=-+
  Constant : Constant  OutDataTypeStr=single
  Constant1 : Constant  Value=0  OutDataTypeStr=single
  Demux : Demux  Outputs=2
  Mux : Mux  Inputs=2
  Mux1 : Mux  Inputs=2
  Relational Operator : RelationalOperator  Operator=<=  OutDataTypeStr=boolean  RndMeth=Simplest  InputSameDT=off
  Switch : Switch  Criteria=u2 > Threshold  SaturateOnIntegerOverflow=off  InputSameDT=off
  T1 : Outport
  T2 : Outport  Port=2
  wires:
  T6_m/1 -> Add1/2, Relational Operator/1
  delta/1 -> Add/1, Add1/1, Relational Operator/2
  Relational Operator/1 -> Switch/2
  Constant/1 -> Mux/1
  Constant1/1 -> Mux/2
  Mux/1 -> Switch/1
  T4_m/1 -> Add/2
  Add/1 -> Mux1/1
  Add1/1 -> Mux1/2
  Mux1/1 -> Switch/3
  Switch/1 -> Demux/1
  Demux/1 -> T1/1
  Demux/2 -> T2/1

== system PMSM_Simulation/Subsystem/Subsystem/SVM_PU/T1_T2_Calc/Subsystem2/If Action Subsystem2/If Action Subsystem3 ==
  T4_m : Inport
  T6_m : Inport  Port=2
  delta : Inport  Port=3
  Action Port : ActionPort  ActionPortLabel=else
  Add : Sum
  Add1 : Sum  Inputs=-+
  Constant : Constant  OutDataTypeStr=single
  Constant1 : Constant  Value=0  OutDataTypeStr=single
  Demux : Demux  Outputs=2
  Mux : Mux  Inputs=2
  Mux1 : Mux  Inputs=2
  Relational Operator : RelationalOperator  Operator=<=  OutDataTypeStr=boolean  RndMeth=Simplest  InputSameDT=off
  Switch : Switch  Criteria=u2 > Threshold  SaturateOnIntegerOverflow=off  InputSameDT=off
  T1 : Outport
  T2 : Outport  Port=2
  wires:
  Mux1/1 -> Switch/3
  delta/1 -> Add/1, Add1/1, Relational Operator/2
  Add1/1 -> Mux1/2
  Mux/1 -> Switch/1
  Relational Operator/1 -> Switch/2
  Switch/1 -> Demux/1
  Constant1/1 -> Mux/2
  Add/1 -> Mux1/1
  Constant/1 -> Mux/1
  T4_m/1 -> Add1/2, Relational Operator/1
  T6_m/1 -> Add/2
  Demux/2 -> T1/1
  Demux/1 -> T2/1

== system PMSM_Simulation/Subsystem/Subsystem/Subsystem2/Subsystem/Tavon_Calc/ia/If Action Subsystem ==
  Phase_Dyc : Inport
  uIgbt : Inport  Port=2
  uDde : Inport  Port=3
  uDcLink : Inport  Port=4
  Action Port : ActionPort  ActionPortLabel=if(u1 == 1)
  Add : Sum  Inputs=-+
  Add1 : Sum  Inputs=+-
  Add2 : Sum  Inputs=--+
  Constant : Constant  OutDataTypeStr=single
  Divide : Product  Inputs=*/
  Product : Product
  Product1 : Product
  "dycCorr " : Outport
  wires:
  Phase_Dyc/1 -> Product/1, Add/1
  uIgbt/1 -> Product/2, Add2/1
  uDde/1 -> Add2/2, Product1/2
  Add/1 -> Product1/1
  Constant/1 -> Add/2
  Product/1 -> Add1/1
  Product1/1 -> Add1/2
  uDcLink/1 -> Add2/3
  Add1/1 -> Divide/1
  Add2/1 -> Divide/2
  Divide/1 -> "dycCorr "/1

== system PMSM_Simulation/Subsystem/Subsystem/Subsystem2/Subsystem/Tavon_Calc/ia/If Action Subsystem1 ==
  Phase_Dyc : Inport
  uIgbt : Inport  Port=2
  uDde : Inport  Port=3
  uDcLink : Inport  Port=4
  Action Port : ActionPort  ActionPortLabel=else
  Add : Sum  Inputs=-+
  Add1 : Sum  Inputs=+-
  Add2 : Sum  Inputs=--+
  Constant : Constant  OutDataTypeStr=single
  Divide : Product  Inputs=*/
  Product : Product
  Product1 : Product
  "dycCorr " : Outport
  wires:
  Phase_Dyc/1 -> Product/1, Add/1
  uDde/1 -> Add2/1, Product/2
  uIgbt/1 -> Add2/2, Product1/2
  Add/1 -> Product1/1
  Constant/1 -> Add/2
  Product/1 -> Add1/1
  Product1/1 -> Add1/2
  uDcLink/1 -> Add2/3
  Add1/1 -> Divide/1
  Add2/1 -> Divide/2
  Divide/1 -> "dycCorr "/1

== system PMSM_Simulation/Subsystem/Subsystem/Subsystem2/Subsystem/Tavon_Calc/ia/uDdeCalc ==
  iPhaseAbs : Inport
  Compare To Constant : simulink/Logic and Bit Operations/Compare To Constant  relop=<  const=VfDeadCompen_ISttrDdeThdSwt_A  OutDataTypeStr=boolean
  From : From
  From1 : From
  Goto : Goto
  If : If  IfExpression=u1 == 1
  If Action Subsystem : Subsystem  TreatAsAtomicUnit=on
  If Action Subsystem1 : Subsystem  TreatAsAtomicUnit=on
  Merge : Merge
  uDde : Outport
  wires:
  iPhaseAbs/1 -> Goto/1, Compare To Constant/1
  If/2 -> If Action Subsystem1/Action
  Merge/1 -> uDde/1
  If/1 -> If Action Subsystem/Action
  If Action Subsystem/1(UDde) -> Merge/1
  Compare To Constant/1 -> If/1
  If Action Subsystem1/1(UDde) -> Merge/2
  From1/1 -> If Action Subsystem/1(iPhaseAbs)
  From/1 -> If Action Subsystem1/1(iPhaseAbs)

== system PMSM_Simulation/Subsystem/Subsystem/Subsystem2/Subsystem/Tavon_Calc/ia/uIgbtCalc ==
  iPhaseAbs : Inport
  Compare To Constant : simulink/Logic and Bit Operations/Compare To Constant  relop=<  const=VfDeadCompen_ISttrIgbtThdSwt_A  OutDataTypeStr=boolean
  If : If  IfExpression=u1 == 0
  If Action Subsystem : Subsystem  TreatAsAtomicUnit=on
  If Action Subsystem1 : Subsystem  TreatAsAtomicUnit=on
  Merge : Merge
  uIgbt : Outport
  wires:
  iPhaseAbs/1 -> Compare To Constant/1, [B]
  If/2 -> If Action Subsystem1/Action
  Merge/1 -> uIgbt/1
  If/1 -> If Action Subsystem/Action
  If Action Subsystem/1(uIgbt) -> Merge/1
  Compare To Constant/1 -> If/1
  If Action Subsystem1/1(uIgbt) -> Merge/2
  [B] -> If Action Subsystem/1(iPhaseAbs)
  [B] -> If Action Subsystem1/1(iPhaseAbs)

== system PMSM_Simulation/Subsystem/Subsystem/Subsystem2/Subsystem/Tavon_Calc/ia1/If Action Subsystem ==
  Phase_Dyc : Inport
  uIgbt : Inport  Port=2
  uDde : Inport  Port=3
  uDcLink : Inport  Port=4
  Action Port : ActionPort  ActionPortLabel=if(u1 == 1)
  Add : Sum  Inputs=-+
  Add1 : Sum  Inputs=+-
  Add2 : Sum  Inputs=--+
  Constant : Constant  OutDataTypeStr=single
  Divide : Product  Inputs=*/
  Product : Product
  Product1 : Product
  "dycCorr " : Outport
  wires:
  Phase_Dyc/1 -> Product/1, Add/1
  uIgbt/1 -> Product/2, Add2/1
  uDde/1 -> Add2/2, Product1/2
  Add/1 -> Product1/1
  Constant/1 -> Add/2
  Product/1 -> Add1/1
  Product1/1 -> Add1/2
  uDcLink/1 -> Add2/3
  Add1/1 -> Divide/1
  Add2/1 -> Divide/2
  Divide/1 -> "dycCorr "/1

== system PMSM_Simulation/Subsystem/Subsystem/Subsystem2/Subsystem/Tavon_Calc/ia1/If Action Subsystem1 ==
  Phase_Dyc : Inport
  uIgbt : Inport  Port=2
  uDde : Inport  Port=3
  uDcLink : Inport  Port=4
  Action Port : ActionPort  ActionPortLabel=else
  Add : Sum  Inputs=-+
  Add1 : Sum  Inputs=+-
  Add2 : Sum  Inputs=--+
  Constant : Constant  OutDataTypeStr=single
  Divide : Product  Inputs=*/
  Product : Product
  Product1 : Product
  "dycCorr " : Outport
  wires:
  Phase_Dyc/1 -> Product/1, Add/1
  uDde/1 -> Add2/1, Product/2
  uIgbt/1 -> Add2/2, Product1/2
  Add/1 -> Product1/1
  Constant/1 -> Add/2
  Product/1 -> Add1/1
  Product1/1 -> Add1/2
  uDcLink/1 -> Add2/3
  Add1/1 -> Divide/1
  Add2/1 -> Divide/2
  Divide/1 -> "dycCorr "/1

== system PMSM_Simulation/Subsystem/Subsystem/Subsystem2/Subsystem/Tavon_Calc/ia1/uDdeCalc ==
  iPhaseAbs : Inport
  Compare To Constant : simulink/Logic and Bit Operations/Compare To Constant  relop=<  const=VfDeadCompen_ISttrDdeThdSwt_A  OutDataTypeStr=boolean
  From : From
  From1 : From
  Goto : Goto
  If : If  IfExpression=u1 == 1
  If Action Subsystem : Subsystem  TreatAsAtomicUnit=on
  If Action Subsystem1 : Subsystem  TreatAsAtomicUnit=on
  Merge : Merge
  uDde : Outport
  wires:
  iPhaseAbs/1 -> Goto/1, Compare To Constant/1
  If/2 -> If Action Subsystem1/Action
  Merge/1 -> uDde/1
  If/1 -> If Action Subsystem/Action
  If Action Subsystem/1(UDde) -> Merge/1
  Compare To Constant/1 -> If/1
  If Action Subsystem1/1(UDde) -> Merge/2
  From1/1 -> If Action Subsystem/1(iPhaseAbs)
  From/1 -> If Action Subsystem1/1(iPhaseAbs)

== system PMSM_Simulation/Subsystem/Subsystem/Subsystem2/Subsystem/Tavon_Calc/ia1/uIgbtCalc ==
  iPhaseAbs : Inport
  Compare To Constant : simulink/Logic and Bit Operations/Compare To Constant  relop=<  const=VfDeadCompen_ISttrIgbtThdSwt_A  OutDataTypeStr=boolean
  If : If  IfExpression=u1 == 0
  If Action Subsystem : Subsystem  TreatAsAtomicUnit=on
  If Action Subsystem1 : Subsystem  TreatAsAtomicUnit=on
  Merge : Merge
  uIgbt : Outport
  wires:
  iPhaseAbs/1 -> Compare To Constant/1, [B]
  If/2 -> If Action Subsystem1/Action
  Merge/1 -> uIgbt/1
  If/1 -> If Action Subsystem/Action
  If Action Subsystem/1(uIgbt) -> Merge/1
  Compare To Constant/1 -> If/1
  If Action Subsystem1/1(uIgbt) -> Merge/2
  [B] -> If Action Subsystem/1(iPhaseAbs)
  [B] -> If Action Subsystem1/1(iPhaseAbs)

== system PMSM_Simulation/Subsystem/Subsystem/Subsystem2/Subsystem/Tavon_Calc/ia2/If Action Subsystem ==
  Phase_Dyc : Inport
  uIgbt : Inport  Port=2
  uDde : Inport  Port=3
  uDcLink : Inport  Port=4
  Action Port : ActionPort  ActionPortLabel=if(u1 == 1)
  Add : Sum  Inputs=-+
  Add1 : Sum  Inputs=+-
  Add2 : Sum  Inputs=--+
  Constant : Constant  OutDataTypeStr=single
  Divide : Product  Inputs=*/
  Product : Product
  Product1 : Product
  "dycCorr " : Outport
  wires:
  Phase_Dyc/1 -> Product/1, Add/1
  uIgbt/1 -> Product/2, Add2/1
  uDde/1 -> Add2/2, Product1/2
  Add/1 -> Product1/1
  Constant/1 -> Add/2
  Product/1 -> Add1/1
  Product1/1 -> Add1/2
  uDcLink/1 -> Add2/3
  Add1/1 -> Divide/1
  Add2/1 -> Divide/2
  Divide/1 -> "dycCorr "/1

== system PMSM_Simulation/Subsystem/Subsystem/Subsystem2/Subsystem/Tavon_Calc/ia2/If Action Subsystem1 ==
  Phase_Dyc : Inport
  uIgbt : Inport  Port=2
  uDde : Inport  Port=3
  uDcLink : Inport  Port=4
  Action Port : ActionPort  ActionPortLabel=else
  Add : Sum  Inputs=-+
  Add1 : Sum  Inputs=+-
  Add2 : Sum  Inputs=--+
  Constant : Constant  OutDataTypeStr=single
  Divide : Product  Inputs=*/
  Product : Product
  Product1 : Product
  "dycCorr " : Outport
  wires:
  Phase_Dyc/1 -> Product/1, Add/1
  uDde/1 -> Add2/1, Product/2
  uIgbt/1 -> Add2/2, Product1/2
  Add/1 -> Product1/1
  Constant/1 -> Add/2
  Product/1 -> Add1/1
  Product1/1 -> Add1/2
  uDcLink/1 -> Add2/3
  Add1/1 -> Divide/1
  Add2/1 -> Divide/2
  Divide/1 -> "dycCorr "/1

== system PMSM_Simulation/Subsystem/Subsystem/Subsystem2/Subsystem/Tavon_Calc/ia2/uDdeCalc ==
  iPhaseAbs : Inport
  Compare To Constant : simulink/Logic and Bit Operations/Compare To Constant  relop=<  const=VfDeadCompen_ISttrDdeThdSwt_A  OutDataTypeStr=boolean
  From : From
  From1 : From
  Goto : Goto
  If : If  IfExpression=u1 == 1
  If Action Subsystem : Subsystem  TreatAsAtomicUnit=on
  If Action Subsystem1 : Subsystem  TreatAsAtomicUnit=on
  Merge : Merge
  uDde : Outport
  wires:
  iPhaseAbs/1 -> Goto/1, Compare To Constant/1
  If/2 -> If Action Subsystem1/Action
  Merge/1 -> uDde/1
  If/1 -> If Action Subsystem/Action
  If Action Subsystem/1(UDde) -> Merge/1
  Compare To Constant/1 -> If/1
  If Action Subsystem1/1(UDde) -> Merge/2
  From1/1 -> If Action Subsystem/1(iPhaseAbs)
  From/1 -> If Action Subsystem1/1(iPhaseAbs)

== system PMSM_Simulation/Subsystem/Subsystem/Subsystem2/Subsystem/Tavon_Calc/ia2/uIgbtCalc ==
  iPhaseAbs : Inport
  Compare To Constant : simulink/Logic and Bit Operations/Compare To Constant  relop=<  const=VfDeadCompen_ISttrIgbtThdSwt_A  OutDataTypeStr=boolean
  If : If  IfExpression=u1 == 0
  If Action Subsystem : Subsystem  TreatAsAtomicUnit=on
  If Action Subsystem1 : Subsystem  TreatAsAtomicUnit=on
  Merge : Merge
  uIgbt : Outport
  wires:
  iPhaseAbs/1 -> Compare To Constant/1, [B]
  If/2 -> If Action Subsystem1/Action
  Merge/1 -> uIgbt/1
  If/1 -> If Action Subsystem/Action
  If Action Subsystem/1(uIgbt) -> Merge/1
  Compare To Constant/1 -> If/1
  If Action Subsystem1/1(uIgbt) -> Merge/2
  [B] -> If Action Subsystem/1(iPhaseAbs)
  [B] -> If Action Subsystem1/1(iPhaseAbs)

== system PMSM_Simulation/Subsystem/Subsystem/Subsystem2/Subsystem2/Subsystem3/Subsystem2/Subsystem ==
  VfPwmFreq_Hz : Inport
  Add5 : Sum
  KfDeadCompen_CpPeriodTimesT_NULL : Constant  Value=KfDeadCompen_CpPeriodTimesT_NULL  OutDataTypeStr=single
  KfMDCC_InvParkCpPeriodTimesT_NULL : Constant  Value=KfMDCC_InvParkCpPeriodTimesT_NULL
  Product1 : Product
  TimeComp : Outport
  wires:
  KfMDCC_InvParkCpPeriodTimesT_NULL/1 -> Add5/2
  KfDeadCompen_CpPeriodTimesT_NULL/1 -> Add5/1
  VfPwmFreq_Hz/1 -> Product1/2
  Product1/1 -> TimeComp/1
  Add5/1 -> Product1/1

== system PMSM_Simulation/Subsystem/Subsystem/DeadComp_Sys/Subsystem/Tavon_Calc/ia/uDdeCalc/If Action Subsystem ==
  iPhaseAbs : Inport
  Action Port : ActionPort
  Add : Sum
  Constant : Constant  Value=VfDeadCompen_uDdeISttrLo_V
  Constant1 : Constant  Value=VfDeadCompen_rDdeISttrLo_R
  Product : Product
  UDde : Outport
  wires:
  Constant/1 -> Add/1
  Constant1/1 -> Product/1
  iPhaseAbs/1 -> Product/2
  Product/1 -> Add/2
  Add/1 -> UDde/1

== system PMSM_Simulation/Subsystem/Subsystem/DeadComp_Sys/Subsystem/Tavon_Calc/ia/uDdeCalc/If Action Subsystem1 ==
  iPhaseAbs : Inport
  Action Port : ActionPort
  Add : Sum
  Constant : Constant  Value=VfDeadCompen_uDdeISttrHi_V
  Constant1 : Constant  Value=VfDeadCompen_rDdeISttrHi_R
  Product : Product
  UDde : Outport
  wires:
  iPhaseAbs/1 -> Product/2
  Constant/1 -> Add/1
  Add/1 -> UDde/1
  Constant1/1 -> Product/1
  Product/1 -> Add/2

== system PMSM_Simulation/Subsystem/Subsystem/DeadComp_Sys/Subsystem/Tavon_Calc/ia/uIgbtCalc/If Action Subsystem ==
  iPhaseAbs : Inport
  Action Port : ActionPort
  Add : Sum
  Constant : Constant  Value=VfDeadCompen_uIgbtISttrLo_V
  Constant1 : Constant  Value=VfDeadCompen_rIgbtISttrLo_R
  Product : Product
  uIgbt : Outport
  wires:
  Constant/1 -> Add/1
  Constant1/1 -> Product/1
  iPhaseAbs/1 -> Product/2
  Product/1 -> Add/2
  Add/1 -> uIgbt/1

== system PMSM_Simulation/Subsystem/Subsystem/DeadComp_Sys/Subsystem/Tavon_Calc/ia/uIgbtCalc/If Action Subsystem1 ==
  iPhaseAbs : Inport
  Action Port : ActionPort
  Add : Sum
  Constant : Constant  Value=VfDeadCompen_uIgbtISttrHi_V
  Constant1 : Constant  Value=VfDeadCompen_rIgbtISttrHi_R
  Product : Product
  uIgbt : Outport
  wires:
  iPhaseAbs/1 -> Product/2
  Constant/1 -> Add/1
  Add/1 -> uIgbt/1
  Constant1/1 -> Product/1
  Product/1 -> Add/2

== system PMSM_Simulation/Subsystem/Subsystem/DeadComp_Sys/Subsystem/Tavon_Calc/ia1/uDdeCalc/If Action Subsystem ==
  iPhaseAbs : Inport
  Action Port : ActionPort
  Add : Sum
  Constant : Constant  Value=VfDeadCompen_uDdeISttrLo_V
  Constant1 : Constant  Value=VfDeadCompen_rDdeISttrLo_R
  Product : Product
  UDde : Outport
  wires:
  Constant/1 -> Add/1
  Constant1/1 -> Product/1
  iPhaseAbs/1 -> Product/2
  Product/1 -> Add/2
  Add/1 -> UDde/1

== system PMSM_Simulation/Subsystem/Subsystem/DeadComp_Sys/Subsystem/Tavon_Calc/ia1/uDdeCalc/If Action Subsystem1 ==
  iPhaseAbs : Inport
  Action Port : ActionPort
  Add : Sum
  Constant : Constant  Value=VfDeadCompen_uDdeISttrHi_V
  Constant1 : Constant  Value=VfDeadCompen_rDdeISttrHi_R
  Product : Product
  UDde : Outport
  wires:
  iPhaseAbs/1 -> Product/2
  Constant/1 -> Add/1
  Add/1 -> UDde/1
  Constant1/1 -> Product/1
  Product/1 -> Add/2

== system PMSM_Simulation/Subsystem/Subsystem/DeadComp_Sys/Subsystem/Tavon_Calc/ia1/uIgbtCalc/If Action Subsystem ==
  iPhaseAbs : Inport
  Action Port : ActionPort
  Add : Sum
  Constant : Constant  Value=VfDeadCompen_uIgbtISttrLo_V
  Constant1 : Constant  Value=VfDeadCompen_rIgbtISttrLo_R
  Product : Product
  uIgbt : Outport
  wires:
  Constant/1 -> Add/1
  Constant1/1 -> Product/1
  iPhaseAbs/1 -> Product/2
  Product/1 -> Add/2
  Add/1 -> uIgbt/1

== system PMSM_Simulation/Subsystem/Subsystem/DeadComp_Sys/Subsystem/Tavon_Calc/ia1/uIgbtCalc/If Action Subsystem1 ==
  iPhaseAbs : Inport
  Action Port : ActionPort
  Add : Sum
  Constant : Constant  Value=VfDeadCompen_uIgbtISttrHi_V
  Constant1 : Constant  Value=VfDeadCompen_rIgbtISttrHi_R
  Product : Product
  uIgbt : Outport
  wires:
  iPhaseAbs/1 -> Product/2
  Constant/1 -> Add/1
  Add/1 -> uIgbt/1
  Constant1/1 -> Product/1
  Product/1 -> Add/2

== system PMSM_Simulation/Subsystem/Subsystem/DeadComp_Sys/Subsystem/Tavon_Calc/ia2/uDdeCalc/If Action Subsystem ==
  iPhaseAbs : Inport
  Action Port : ActionPort
  Add : Sum
  Constant : Constant  Value=VfDeadCompen_uDdeISttrLo_V
  Constant1 : Constant  Value=VfDeadCompen_rDdeISttrLo_R
  Product : Product
  UDde : Outport
  wires:
  Constant/1 -> Add/1
  Constant1/1 -> Product/1
  iPhaseAbs/1 -> Product/2
  Product/1 -> Add/2
  Add/1 -> UDde/1

== system PMSM_Simulation/Subsystem/Subsystem/DeadComp_Sys/Subsystem/Tavon_Calc/ia2/uDdeCalc/If Action Subsystem1 ==
  iPhaseAbs : Inport
  Action Port : ActionPort
  Add : Sum
  Constant : Constant  Value=VfDeadCompen_uDdeISttrHi_V
  Constant1 : Constant  Value=VfDeadCompen_rDdeISttrHi_R
  Product : Product
  UDde : Outport
  wires:
  iPhaseAbs/1 -> Product/2
  Constant/1 -> Add/1
  Add/1 -> UDde/1
  Constant1/1 -> Product/1
  Product/1 -> Add/2

== system PMSM_Simulation/Subsystem/Subsystem/DeadComp_Sys/Subsystem/Tavon_Calc/ia2/uIgbtCalc/If Action Subsystem ==
  iPhaseAbs : Inport
  Action Port : ActionPort
  Add : Sum
  Constant : Constant  Value=VfDeadCompen_uIgbtISttrLo_V
  Constant1 : Constant  Value=VfDeadCompen_rIgbtISttrLo_R
  Product : Product
  uIgbt : Outport
  wires:
  Constant/1 -> Add/1
  Constant1/1 -> Product/1
  iPhaseAbs/1 -> Product/2
  Product/1 -> Add/2
  Add/1 -> uIgbt/1
